simulink model "SOC_SOP_SOE_Test_prev"  (R2022b)
settings: Solver=VariableStepAuto  StartTime=0.0  StopTime=7900  RelTol=1e-3
values from neighbouring files (symbols this model uses):
  NumModules = 1.0    [Global_Parameters.sldd]
  NumParallel = 30.0    [Global_Parameters.sldd]
  NumSeries = 24.0    [Global_Parameters.sldd]
settings Model: DataDictionary=Global_Parameters.sldd  Creator=japerez  LastModifiedBy=jgavidia
settings DebuggingCC: ParameterPrecisionLossMsg=none

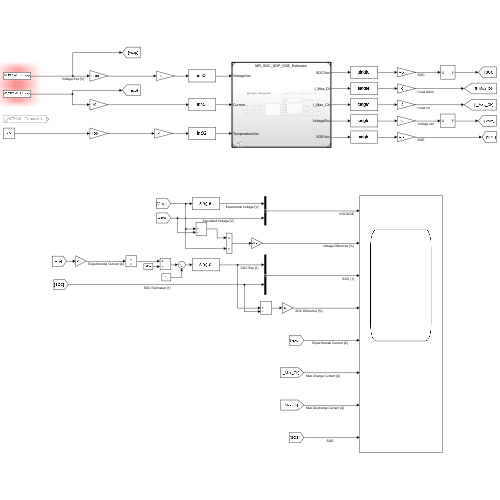
[thumbnail: Simulink's stored preview of the top-level diagram]
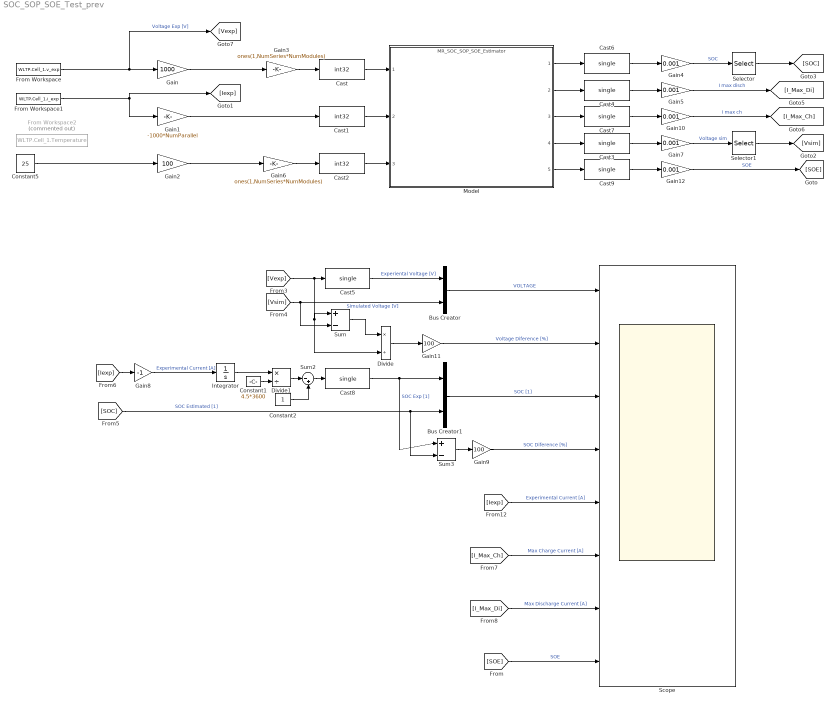
== system SOC_SOP_SOE_Test_prev ==
  Bus Creator : BusCreator  Inputs=2
  Bus Creator1 : BusCreator  Inputs=2
  Cast : DataTypeConversion  OutDataTypeStr=int32  SaturateOnIntegerOverflow=off  RndMeth=Floor
  Cast1 : DataTypeConversion  OutDataTypeStr=int32  SaturateOnIntegerOverflow=off  RndMeth=Floor
  Cast2 : DataTypeConversion  OutDataTypeStr=int32  SaturateOnIntegerOverflow=off  RndMeth=Floor
  Cast{3..9} (7 alike) : DataTypeConversion  OutDataTypeStr=single  SaturateOnIntegerOverflow=off  RndMeth=Floor
  Constant1 : Constant  Value=4.5*3600
  Constant2 : Constant
  Constant5 : Constant  Value=25
  Divide : Product  Inputs=*/
  Divide1 : Product  Inputs=*/
  From Workspace : FromWorkspace  VariableName=WLTP.Cell_1.v_exp
  From Workspace1 : FromWorkspace  VariableName=WLTP.Cell_1.i_exp
  From Workspace2 : FromWorkspace  Commented=on  VariableName=WLTP.Cell_1.Temperature
  Gain : Gain  Gain=1000
  Gain1 : Gain  Gain=-1000*NumParallel
  Gain{4..5,7,10,12} (5 alike) : Gain  Gain=0.001
  Gain11 : Gain  Gain=100
  Gain2 : Gain  Gain=100
  Gain3 : Gain  Gain=ones(1,NumSeries*NumModules)
  Gain6 : Gain  Gain=ones(1,NumSeries*NumModules)
  Gain8 : Gain  Gain=-1
  Gain9 : Gain  Gain=100
  Integrator : Integrator
  Model : ModelReference  ModelNameDialog=MR_SOC_SOP_SOE_Estimator.slx  SimulationMode=Normal  ModelReferenceVersion=1.83
  Scope : Scope  NumInputPorts=8
  Selector : Selector  InputPortWidth=24  IndexOptions=Index vector (dialog)  Indices=1  OutputSizes=1
  Selector1 : Selector  InputPortWidth=24  IndexOptions=Index vector (dialog)  Indices=1  OutputSizes=1
  Sum : Sum  Inputs=|+-
  Sum2 : Sum  Inputs=|-+
  Sum3 : Sum  Inputs=|+-
  wires:
  From Workspace/1 -> [Vexp], Gain/1  "Voltage Exp [V]"
  Gain/1 -> Gain3/1
  Gain3/1 -> Cast/1
  Cast/1 -> Model/1
  Cast1/1 -> Model/2
  Gain1/1 -> Cast1/1
  Gain2/1 -> Gain6/1
  Cast2/1 -> Model/3
  Cast4/1 -> Gain5/1
  Gain6/1 -> Cast2/1
  Gain4/1 -> Selector/1  "SOC"
  Gain5/1 -> [I_Max_Di]  "I max disch"
  Gain10/1 -> [I_Max_Ch]  "I max ch"
  Cast7/1 -> Gain10/1
  Model/3 -> Cast7/1
  Model/1 -> Cast6/1
  Model/2 -> Cast4/1
  Cast3/1 -> Gain7/1
  Model/4 -> Cast3/1
  Gain7/1 -> Selector1/1  "Voltage sim"
  Selector1/1 -> [Vsim]
  From Workspace1/1 -> Gain1/1, [Iexp]
  [Vsim] -> Sum/2, Bus Creator/2  "Simulated Voltage [V]"
  Sum/1 -> Divide/1
  Divide/1 -> Gain11/1
  Bus Creator/1 -> Scope/1  "VOLTAGE"
  [Vexp] -> Divide/2, Sum/1, Cast5/1
  Cast5/1 -> Bus Creator/1  "Experiental Voltage [V]"
  Selector/1 -> [SOC]
  Cast8/1 -> Sum3/1, Bus Creator1/1  "SOC Exp [1]"
  Divide1/1 -> Sum2/1
  Sum2/1 -> Cast8/1
  [Iexp] -> Gain8/1
  Gain8/1 -> Integrator/1  "Experimental Current [A]"
  Constant2/1 -> Sum2/2
  Constant1/1 -> Divide1/2
  [SOC] -> Bus Creator1/2, Sum3/2  "SOC Estimated [1]"
  Integrator/1 -> Divide1/1
  Bus Creator1/1 -> Scope/3  "SOC [1]"
  Gain11/1 -> Scope/2  "Voltage Diference [%]"
  Sum3/1 -> Gain9/1
  [I_Max_Ch] -> Scope/6  "Max Charge Current [A]"
  [I_Max_Di] -> Scope/7  "Max Discharge Current [A]"
  [Iexp] -> Scope/5  "Experimental Current [A]"
  Gain9/1 -> Scope/4  "SOC Diference [%]"
  Model/5 -> Cast9/1
  Cast9/1 -> Gain12/1
  Gain12/1 -> [SOE]  "SOE"
  [SOE] -> Scope/8  "SOE"
  Cast6/1 -> Gain4/1
  Constant5/1 -> Gain2/1
